simulink model "echo_model"  (R2023a)
settings: Solver=VariableStepAuto  StartTime=0.0  StopTime=2.0  RelTol=1e-3
libraries: spspowerguiLib x1
settings Model: Creator=86198  LastModifiedBy=86198

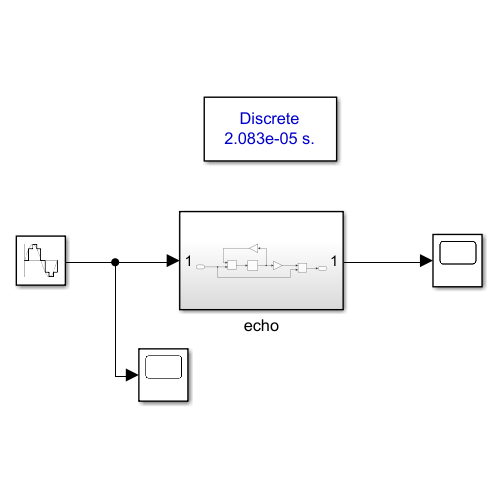
[thumbnail: Simulink's stored preview of the top-level diagram]
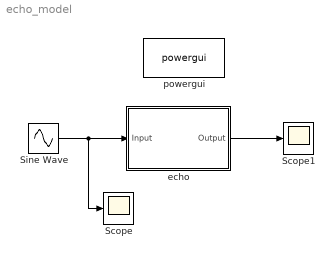
== system echo_model ==
  Scope : Scope
  Scope1 : Scope
  Sine Wave : Sin  Frequency=2*pi*1125  SampleTime=1/48000
  echo : Subsystem
  powergui : spspowerguiLib/powergui  Priority=1  SimulationMode=Discrete  SampleTime=1/48000  frequency=60  Iterations=50  frequencyindice=60  Pbase=100e6  ErrMax=1e-4  UnitsV=kV  UnitsW=MW  buscounter=0  FunctionMessages=off  echomessages=off  EnableUseOfTLC=off  CurrentSourceSwitches=off  DisableSnubberDevices=off  DisableRonSwitches=off  DisableVfSwitches=off  DisplayEquations=off  AutomaticDiscreteSolvers=off  SolverType=Tustin/Backward Euler (TBE)  Interpol=off  ExternalGateDelay=off  methode=off  Ts=100  x0status=blocks  SPID=on  SwTol=0  HookPort=off  NonlinearTolerance=1e-4  nMaxIteration=100  ContinueOnMaxIteration=off  RestoreLinks=warning  ResistiveCurrentMeasurement=off  Frange=[0:2:500]  Ylog=off  Xlog=on  ShowGrid=off  save=off  variable=ZData  structure=0  ZoomFFT=off  StartTime=0.0  cycles=1  DisplayStyle=1  fundamental=60  FreqAxis=off  MaxFrequency=1000  frequencyindicesteady=1  RmsSteady=1  display=off
  wires:
  Sine Wave/1 -> Scope/1, echo/1(Input)
  echo/1(Output) -> Scope1/1

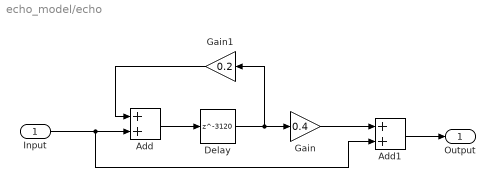
== system echo_model/echo ==
  Input : Inport
  Add : Sum
  Add1 : Sum
  Delay : Delay  DelayLength=3120
  Gain : Gain  Gain=0.4
  Gain1 : Gain  Gain=0.2
  Output : Outport
  wires:
  Add/1 -> Delay/1
  Delay/1 -> Gain1/1, Gain/1
  Gain1/1 -> Add/1
  Gain/1 -> Add1/1
  Input/1 -> Add1/2, Add/2
  Add1/1 -> Output/1
